simulink model "Lab1_DC_Motor_Test"  (R2026a)
settings: Solver=FixedStepDiscrete  StopTime=inf  FixedStep=0.05
libraries: arduinolib x4, arduinosensorlib x1
settings Model: SILPILModeSetting=veronly  ExtModeTrigDuration=2  Creator=chawi  LastModifiedBy=chawi
settings HardwareCC: ProdBitPerInt=16.0  ProdBitPerPointer=16.0  ProdBitPerSizeT=16.0  ProdBitPerPtrDiffT=16.0  ProdWordSize=8.0  ProdHWDeviceType=Atmel->AVR
settings RTWCC: SystemTargetFile=ert.tlc  HardwareBoard=Arduino Uno  TLCOptions=-aInlineSetEventsForThisBaseRateFcn=TLC_FALSE -aSuppressMultiTaskScheduler=TLC_FALSE -aRateBasedStepFcn=1  Toolchain=Arduino AVR  BuildConfiguration=Faster Runs  Description=Embedded Coder
settings ERTTargetCC: ExtModeTransport=3.0  ExtModeAutomaticAllocSize=off  ExtModeStaticAllocSize=250.0  SupportContinuousTime=on  SupportVariableSizeSignals=on

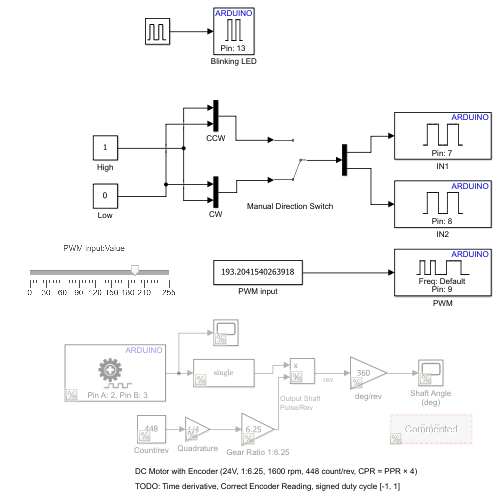
[thumbnail: Simulink's stored preview of the top-level diagram]
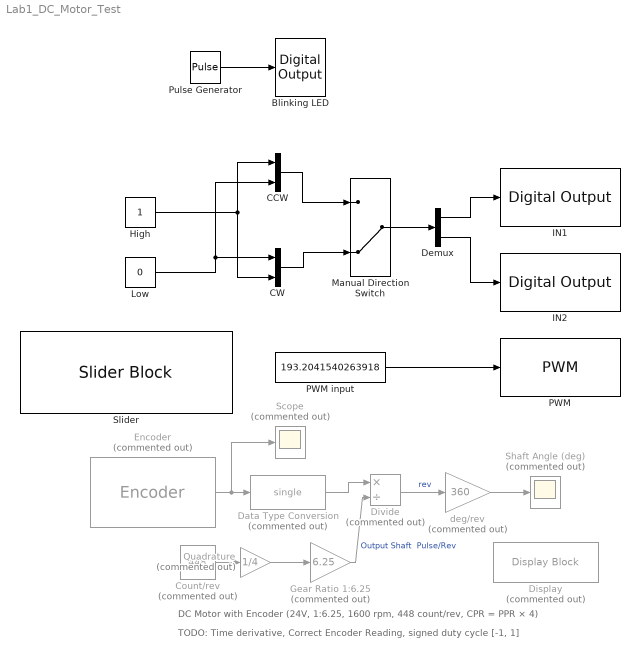
== system Lab1_DC_Motor_Test ==
  note: TODO: Time derivative, Correct Encoder Reading, signed duty cycle [-1, 1]
  note: DC Motor with Encoder (24V, 1:6.25, 1600 rpm, 448 count/rev, CPR = PPR × 4)
  Blinking LED : arduinolib/Digital Output  pinNumber=13  Direction=output  blockPlatform=arduino
  CCW : Mux  Inputs=2
  CW : Mux  Inputs=2
  Count/rev : Constant  Commented=on  Value=448
  Data Type Conversion : DataTypeConversion  Commented=on  OutDataTypeStr=single  SaturateOnIntegerOverflow=off  RndMeth=Floor
  Demux : Demux  Outputs=2
  Display : DisplayBlock  Commented=on  LabelPosition=Hide  Transparency=1  GridColor=[0.502, 0.502, 0.502]
  Divide : Product  Commented=on  Inputs=*/
  Encoder : arduinosensorlib/Encoder  Commented=on  InputA=2  InputB=3  Mode=No reset  SampleTime=-1
  Gear Ratio 1:6.25 : Gain  Commented=on  Gain=6.25
  High : Constant  OutMin=0  OutMax=1  OutDataTypeStr=uint8
  IN1 : arduinolib/Digital Output  pinNumber=7  Direction=output  blockPlatform=arduino
  IN2 : arduinolib/Digital Output  pinNumber=8  Direction=output  blockPlatform=arduino
  Low : Constant  Value=0  OutMin=0  OutMax=1  OutDataTypeStr=uint8
  Manual Direction Switch : ManualSwitch  CurrentSetting=0
  PWM : arduinolib/PWM  pinNumber=9  frequencyType=Default  desiredFrequency=490.2  achievableFrequency=490.2
  PWM input : Constant  Value=193.2041540263918  OutMin=0  OutMax=255  OutDataTypeStr=uint8
  Pulse Generator : DiscretePulseGenerator  PulseType=Time based  Period=1  PulseWidth=50
  Quadrature : Gain  Commented=on  Gain=1/4
  Scope : Scope  Commented=on
      settings: ActiveDisplayYMinimum=-1257.9162206365634  ActiveDisplayYMaximum=523.60648978583447
  Shaft Angle (deg) : Scope  Commented=on
      settings: ActiveDisplayYMinimum=-6135.75  ActiveDisplayYMaximum=681.74999999999989
  Slider : SliderBlock  ScaleMax=255
  deg/rev : Gain  Commented=on  Gain=360
  wires:
  Count/rev/1 -> Quadrature/1
  Gear Ratio 1:6.25/1 -> Divide/2  "Output Shaft  Pulse/Rev"
  Divide/1 -> deg/rev/1  "rev"
  deg/rev/1 -> Shaft Angle (deg)/1
  Pulse Generator/1 -> Blinking LED/1
  CW/1 -> Manual Direction Switch/2
  High/1 -> CCW/1, CW/2
  Low/1 -> CCW/2, CW/1
  CCW/1 -> Manual Direction Switch/1
  Manual Direction Switch/1 -> Demux/1
  Demux/1 -> IN1/1
  Demux/2 -> IN2/1
  PWM input/1 -> PWM/1
  Quadrature/1 -> Gear Ratio 1:6.25/1
  Encoder/1 -> Scope/1, Data Type Conversion/1
  Data Type Conversion/1 -> Divide/1
